simulink model "TestAirCooledPDUAssembly"  (R2025b)
settings: Solver=daessc  StartTime=0.0  StopTime=1200  MaxStep=1  RelTol=1e-3  AbsTol=1e-3
libraries: fl_lib x7, nesl_utility x6, datacenterCompositeLib x1
settings Model: Creator=vikrants  LastModifiedBy=vikrants
settings SolverCC: AutoScaleAbsTol=off  AlgebraicLoopSolver=TrustRegion  MaxZcPerStep=1.0
settings DebuggingCC: UnconnectedInputMsg=warning  UnconnectedOutputMsg=warning  UnconnectedLineMsg=warning  SymbolicDimsDataTypeCodeGenerationDiagnostic=none
settings ModelReferenceCC: EnableRefExpFcnMdlSchedulingChecks=on
settings SFSimCC: CustomCodeUndefinedFunction=UseInterfaceOnly
settings RTWCC: GPUComputeCapability=3.5  DLArmComputeVersion=19.05
settings SimscapeCC: SimscapeLogType=all  SimscapeLogSimulationStatistics=on  SimscapeLogDataHistory=10000.0

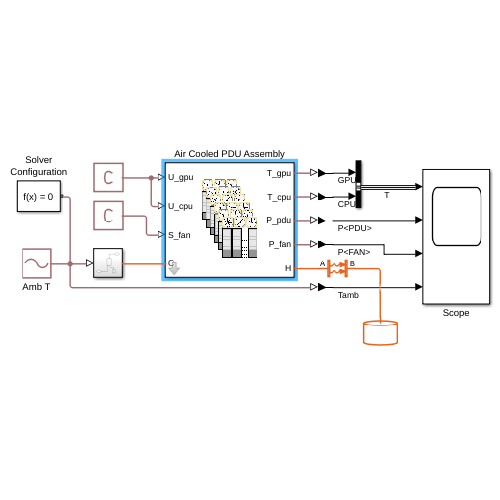
[thumbnail: Simulink's stored preview of the top-level diagram]
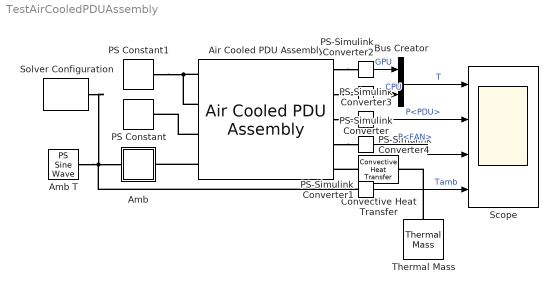
== system TestAirCooledPDUAssembly ==
  Air Cooled PDU Assembly : datacenterCompositeLib/Air Cooled PDU Assembly  nAssembly=3  nRacks=4  nTrays=6  nFans=24  flowVec=[500:200:1300]*0.000472  prDropVec=[7000:250:8000]  fanEffVec=[0.58, 0.60, 0.61, 0.60, 0.59]  refTfan=293  trayMass=10  trayCp=6000  trayThermalR=1e-3  nGPU=4  gpuTDPperDie=1200  gpuIdlePower=300  gpuHBMpower=80  gpuExponent=1.4  gpuHBMutil=0.7  gpuLeakage=1.5  gpuNominalDieT=350  gpuDieThermalC=50  gpuHeatSinkR=1e-3  gpuSurfArea=0.01  gpuAmbientR=1e-3  nCPU=2  cpuTDPperSocket=350  cpuIdlePower=80  cpuExponent=1.1  cpuLeakage=1.5  cpuNominalDieT=350  cpuDieThermalC=50  cpuHeatSinkR=1e-3  cpuSurfArea=0.01  cpuAmbientR=1e-3  initialT=300  htc=10
  Amb : Subsystem
  Amb T : fl_lib/Physical Signals/Sources/PS Sine Wave  amplitude=5 K  bias=270 K  frequency_spec=foundation.enum.frequencySpec.frequencySI  frequency_SI=1/120 Hz  frequency_angular=1 rad/s  phase=0 rad
      settings: InternalSimscapePortConfiguration="{\"Bottom\":[],\"Left\":[],\"Right\":[{\"id\":\"O\",\"label\":\"\",\"type\":\"output\"}],\"Top\":[]}"
  Bus Creator : BusCreator  Inputs=2
  Convective Heat Transfer : fl_lib/Thermal/Thermal Elements/Convective Heat Transfer  thermal_type=foundation.enum.constant_variable.constant  area=0.1 m^2  heat_tr_coeff=4 W/(K*m^2)  min_heat_tr_coeff=1e-3 W/(K*m^2)  T_specify=off  T_priority=None  T=0 K  T_nominal_specify=off  T_nominal_value=1  T_nominal_unit=K  Q_specify=off  Q_priority=None  Q=0 W  Q_nominal_specify=off  Q_nominal_value=1  Q_nominal_unit=W
  PS Constant : fl_lib/Physical Signals/Sources/PS Constant  constant=1
  PS Constant1 : fl_lib/Physical Signals/Sources/PS Constant  constant=.3
  PS-Simulink Converter{,1..4} (5 alike) : nesl_utility/PS-Simulink Converter  PhysicalDomain=network_engine_domain  SubClassName=ps_output  LeftPortType=input  RightPortType=output  PseudoPeriodic=off  Frequencies=[]  VectorFormat=inherit  Unit=inherit  AffineConversion=off
  Scope : Scope  NumInputPorts=4
      settings: ActiveDisplayYMinimum=293.31722069021924  ActiveDisplayYMaximum=302.01292707134837
  Solver Configuration : nesl_utility/Solver Configuration  PhysicalDomain=network_engine_domain  SubClassName=solver  LeftPortType=input  RightPortType=generic  Tones=[]  Harmonics=[]  SimulateNoise=off  Profile=off  UseLocalSampling=off  EnableSwitchedLinearOptims=on  FrequencyDomain=off  UseCCode=off  RelTol=0.001  AbsTol=1e-06  MinStep=1e-09  ToWorkspace=off  RevertToSquareIcSolve=off  NumHomotopyIterations=100  PhasorMode=off  PhasorModeNumHarmonics=1  ConsistencySolver=NEWTON_XTOL_AFTER_FTOL  IndexReductionMethod=DerivativeReplacement  DoDC=off  ResidualTolerance=1e-09  ConsistencyTolSource=GLOBAL  ConsistencyAbsTol=0.001  ConsistencyRelTol=0.001  ConsistencyTolFactor=0.001  UseLocalSolver=off  LocalSolverChoice=NE_BACKWARD_EULER_ADVANCER  ResolveIndetEquations=on  FunctionEvalNumThread=1  LocalSolverSampleTime=0.001  DoFixedCost=off  MaxNonlinIter=3  MaxModeIter=2  ComputeImpulses=off  ImpulseIterations=2  LinearAlgebra=auto  LinearAlgebraNumThread=0  EquationFormulation=NE_TIME_EF  DelaysMemoryBudget=1024  AutomaticFiltering=on  FilteringTimeConstant=0.001  PartitionStorageMethod=AS_NEEDED  PartitionMemoryBudget=1024  PartitionMethod=ROBUST  MultibodyUseLocalSolver=off  MultibodyLocalSolverChoice=ODE1  MultibodyLocalSolverSampleTime=0.001
  Thermal Mass : fl_lib/Thermal/Thermal Elements/Thermal Mass  mass_type=foundation.enum.constant_variable.constant  mass=1000 kg  sp_heat=447 J/(K*kg)  mass_min=1e-6 kg  num_ports=foundation.enum.numPorts2.one  m_specify=off  m_priority=High  m=1 kg  m_nominal_specify=off  m_nominal_value=1  m_nominal_unit=kg  T_specify=off  T_priority=High  T=300 K  T_nominal_specify=off  T_nominal_value=1  T_nominal_unit=K  Q_specify=off  Q_priority=None  Q=0 W  Q_nominal_specify=off  Q_nominal_value=1  Q_nominal_unit=W
  wires:
  PS-Simulink Converter2/1 -> Bus Creator/1  "GPU"
  PS-Simulink Converter/1 -> Bus Creator/2  "CPU"
  Bus Creator/1 -> Scope/1  "T"
  PS-Simulink Converter3/1 -> Scope/2  "P<PDU>"
  PS-Simulink Converter4/1 -> Scope/3  "P<FAN>"
  PS-Simulink Converter1/1 -> Scope/4  "Tamb"
  connections:
  Amb T/RConn1 -- Solver Configuration/RConn1 -- PS-Simulink Converter1/LConn1 -- Amb/LConn1
  Air Cooled PDU Assembly/LConn3 -- PS Constant/RConn1
  PS Constant1/RConn1 -- Air Cooled PDU Assembly/LConn1 -- Air Cooled PDU Assembly/LConn2
  Air Cooled PDU Assembly/LConn4 -- Amb/RConn1
  Air Cooled PDU Assembly/RConn1 -- PS-Simulink Converter2/LConn1
  Air Cooled PDU Assembly/RConn2 -- PS-Simulink Converter/LConn1
  Air Cooled PDU Assembly/RConn3 -- PS-Simulink Converter3/LConn1
  Air Cooled PDU Assembly/RConn4 -- PS-Simulink Converter4/LConn1
  Convective Heat Transfer/LConn1 -- Air Cooled PDU Assembly/RConn5
  Thermal Mass/LConn1 -- Convective Heat Transfer/RConn1

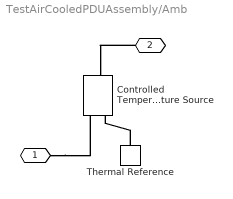
== system TestAirCooledPDUAssembly/Amb ==
  Controlled Temperature Source : fl_lib/Thermal/Thermal Sources/Controlled Temperature Source
  Thermal Reference : fl_lib/Thermal/Thermal Elements/Thermal Reference
  " " : PMIOPort  Side=Left
  "  " : PMIOPort  Port=2  Side=Right
  connections:
  Thermal Reference/LConn1 -- Controlled Temperature Source/RConn2
  " "/RConn1 -- Controlled Temperature Source/RConn1
  "  "/RConn1 -- Controlled Temperature Source/LConn1
